simulink model "NAfinal"  (R2019a)
settings: Solver=ode4  StartTime=0.0  StopTime=2.0  FixedStep=0.0005  RelTol=1e-3
undefined symbols (not defined in the file): den1, den3, in, Kd, Kp, Ldel, Lp, Lpi, num1, num3
settings Model: Creator=xde12  LastModifiedBy=xde12

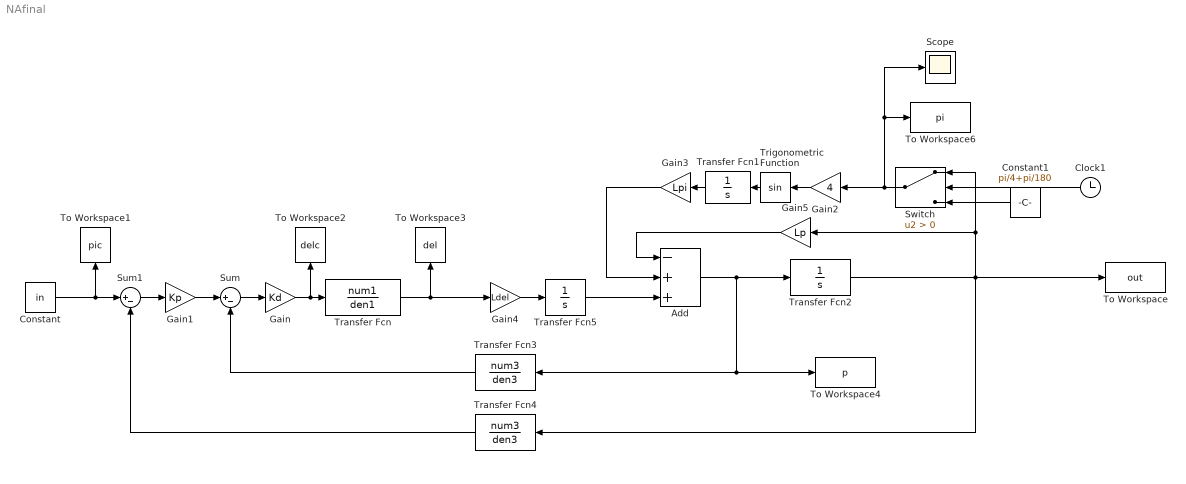
== system NAfinal ==
  Add : Sum  Inputs=-++
  Clock1 : Clock
  Constant : Constant  Value=in
  Constant1 : Constant  Value=pi/4+pi/180
  Gain : Gain  Gain=Kd
  Gain1 : Gain  Gain=Kp
  Gain2 : Gain  Gain=4
  Gain3 : Gain  Gain=Lpi
  Gain4 : Gain  Gain=Ldel
  Gain5 : Gain  Gain=Lp
  Scope : Scope
  Sum : Sum  Inputs=|+-
  Sum1 : Sum  Inputs=|+-
  Switch : Switch  Criteria=u2 > Threshold
  To Workspace : ToWorkspace  VariableName=out  SaveFormat=Structure With Time  SampleTime=-1
  To Workspace1 : ToWorkspace  VariableName=pic  SaveFormat=Structure With Time  SampleTime=-1
  To Workspace2 : ToWorkspace  VariableName=delc  SaveFormat=Structure With Time  SampleTime=-1
  To Workspace3 : ToWorkspace  VariableName=del  SaveFormat=Structure With Time  SampleTime=-1
  To Workspace4 : ToWorkspace  VariableName=p  SaveFormat=Structure With Time  SampleTime=-1
  To Workspace6 : ToWorkspace  VariableName=pi  SaveFormat=Structure With Time  SampleTime=-1
  Transfer Fcn : TransferFcn  Numerator=num1  Denominator=den1
  Transfer Fcn1 : TransferFcn  Denominator=[1 0]
  Transfer Fcn2 : TransferFcn  Denominator=[1 0]
  Transfer Fcn3 : TransferFcn  Numerator=num3  Denominator=den3
  Transfer Fcn4 : TransferFcn  Numerator=num3  Denominator=den3
  Transfer Fcn5 : TransferFcn  Denominator=[1 0]
  Trigonometric Function : Trigonometry
  wires:
  Sum1/1 -> Gain1/1
  Gain1/1 -> Sum/1
  Sum/1 -> Gain/1
  Gain/1 -> To Workspace2/1, Transfer Fcn/1
  Transfer Fcn2/1 -> To Workspace/1, Transfer Fcn4/1, Switch/1, Gain5/1
  Transfer Fcn3/1 -> Sum/2
  Transfer Fcn4/1 -> Sum1/2
  Transfer Fcn/1 -> Gain4/1, To Workspace3/1
  Constant/1 -> To Workspace1/1, Sum1/1
  Gain2/1 -> Trigonometric Function/1
  Constant1/1 -> Switch/3
  Clock1/1 -> Switch/2
  Switch/1 -> Scope/1, To Workspace6/1, Gain2/1
  Gain4/1 -> Transfer Fcn5/1
  Transfer Fcn1/1 -> Gain3/1
  Trigonometric Function/1 -> Transfer Fcn1/1
  Add/1 -> To Workspace4/1, Transfer Fcn3/1, Transfer Fcn2/1
  Transfer Fcn5/1 -> Add/3
  Gain5/1 -> Add/1
  Gain3/1 -> Add/2
